simulink model "MinSegBusTestHarnessFloat08"  (R2014a)
settings: Solver=FixedStepDiscrete  SolverMode=SingleTasking  StartTime=0.0  StopTime=inf  FixedStep=.05  RelTol=1e-3
settings Model: SimulationMode=external  ExtModeTrigDuration=2  Creator=Alec  LastModifiedBy=Brian
settings OptimizationCC: ExpressionDepthLimit=2147483647  OptimizeModelRefInitCode=on  LifeSpan=1
settings DebuggingCC: UnderspecifiedInitializationDetection=Classic  SolverPrmCheckMsg=none  StateNameClashWarn=warning
settings HardwareCC: ProdBitPerInt=16  ProdBitPerPointer=8  ProdIntDivRoundTo=Zero  ProdEndianess=LittleEndian  ProdWordSize=8  ProdHWDeviceType=Atmel->AVR
settings RTWCC: SystemTargetFile=realtime.tlc  GenerateMakefile=off  TemplateMakefile=realtime.tmf  Description=Real-Time Toolbox  RTWVerbose=off  ProcessScript=realtime_make_rtw_hook
settings CodeAppCC: CustomSymbolStrType=$N$R$M  InternalIdentifier=Classic
settings STFCustomTargetCC: TargetLibSuffix=.a  GenerateSampleERTMain=on  ConcurrentExecutionCompliant=off  GeneratePreprocessorConditionals=Use local settings  ERTCustomFileBanners=on  SupportNonInlinedSFcns=off  SupportVariableSizeSignals=on  MATLABClassNameForMDSCustomization=Simulink.SoftwareTarget.ERTCustomization  GRTInterface=off  SystemTargetFile=realtime.tlc
settings ERTTargetCC: CombineOutputUpdateFcns=off  SupportContinuousTime=on  SupportVariableSizeSignals=on  ExtModeTransport=3  ExtModeMexFile=ext_serial_win32_comm  ExtModeMexArgs=0 1 9600  ERTSrcFileBannerTemplate=realtime_code_template.cgt  ERTHdrFileBannerTemplate=realtime_code_template.cgt  ERTDataSrcFileTemplate=realtime_code_template.cgt  ERTDataHdrFileTemplate=realtime_code_template.cgt  ERTCustomFileTemplate=realtime_file_process.tlc

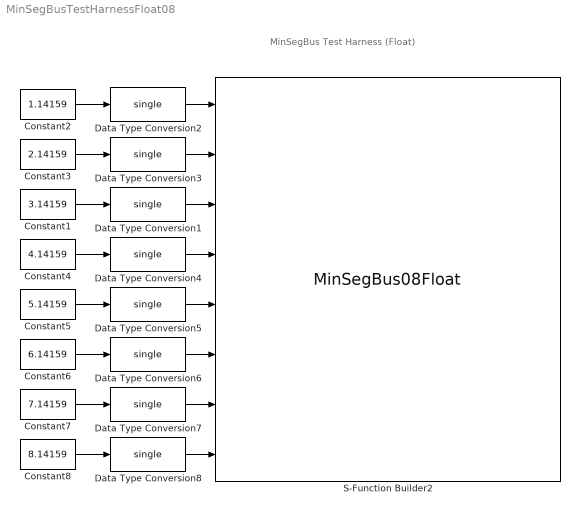
== system MinSegBusTestHarnessFloat08 ==
  note: MinSegBus Test Harness
      | (Float)
  Constant1 : Constant  Value=3.14159
  Constant2 : Constant  Value=1.14159
  Constant3 : Constant  Value=2.14159
  Constant4 : Constant  Value=4.14159
  Constant5 : Constant  Value=5.14159
  Constant6 : Constant  Value=6.14159
  Constant7 : Constant  Value=7.14159
  Constant8 : Constant  Value=8.14159
  Data Type Conversion{1..8} (8 alike) : DataTypeConversion  OutDataTypeStr=single
  S-Function Builder2 : S-Function  InitFcn=try, set_param(gcb,'FunctionName','MinSegBus08Float'), end  FunctionName=MinSegBus08Float  Parameters=int8(4)  SFunctionModules=MinSegBus08Float_wrapper  EnableBusSupport=off  mask(S-Function Builder){}
      mask help: Simulink:masks:SFunctionBuilder_MD
      mask init:
      | val = [[.9  0.75 0.75 1 1 .9 .9 1]',[1 1 0.75 0.75 .9 .9 1 .9]'];try , sys = get_param(gcb,'SfunBuilderFcnName');if isempty(sys), sys = get_param(gcb,'FunctionName'); end,catch, sys = get_param(gcb,'FunctionName'); end
      settings: CopyFcn=set_param(gcbh,'LinkStatus','none')  PreSaveFcn=try, set_param(gcb,'FunctionName','MinSegBus08Float'), end  OpenFcn=sfunctionwizard(gcbh)
      mask Display: plot(val(:,1),val(:,2)),disp(sys), port_label('input',1,'float_01'), port_label('input',2,'float_02'), port_label('input',3,'float_03'), port_label('input',4,'float_04'), port_label('input',5,'float_05'), port_label('input',6,'float_06'), port_label('input',7,'float_07'), port_label('input',8,'float_08')
  wires:
  Constant2/1 -> Data Type Conversion2/1
  Data Type Conversion2/1 -> S-Function Builder2/1
  Constant3/1 -> Data Type Conversion3/1
  Data Type Conversion3/1 -> S-Function Builder2/2
  Constant1/1 -> Data Type Conversion1/1
  Data Type Conversion1/1 -> S-Function Builder2/3
  Constant4/1 -> Data Type Conversion4/1
  Data Type Conversion4/1 -> S-Function Builder2/4
  Data Type Conversion5/1 -> S-Function Builder2/5
  Constant5/1 -> Data Type Conversion5/1
  Constant6/1 -> Data Type Conversion6/1
  Data Type Conversion6/1 -> S-Function Builder2/6
  Data Type Conversion7/1 -> S-Function Builder2/7
  Constant7/1 -> Data Type Conversion7/1
  Constant8/1 -> Data Type Conversion8/1
  Data Type Conversion8/1 -> S-Function Builder2/8
